simulink model "Analyse_Data_LORD"  (R2019b)
settings: Solver=FixedStepAuto  StartTime=0.0  StopTime=6488  FixedStep=0.01  RelTol=1e-3
settings Model: Creator=ReneB  LastModifiedBy=Rene Budich
settings SFSimCC: CustomCodeUndefinedFunction=UseInterfaceOnly

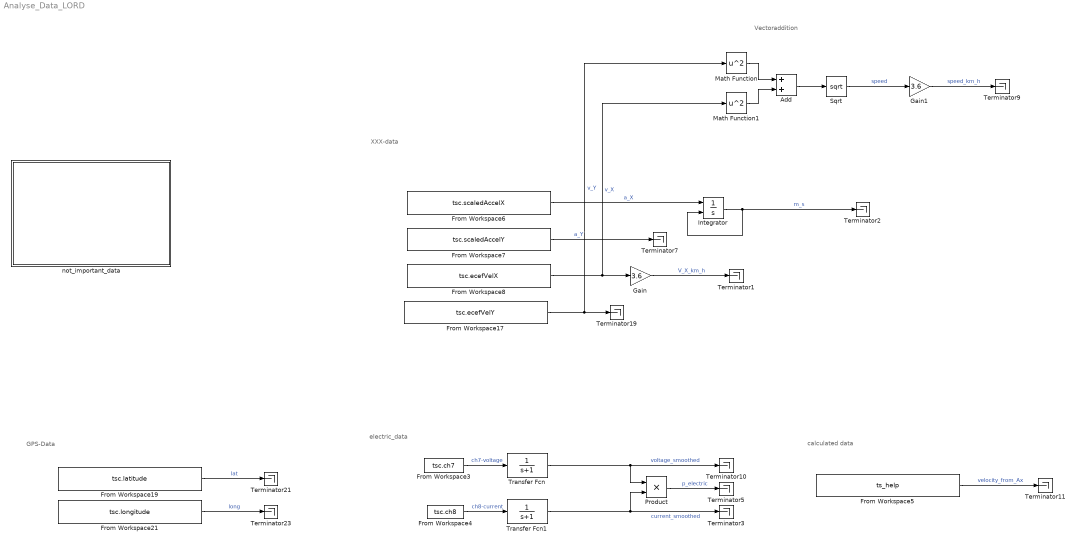
== system Analyse_Data_LORD ==
  note: Vectoraddition
  note: GPS-Data
  note: electric_data
  note: calculated data
  note: XXX-data
  Add : Sum
  From Workspace17 : FromWorkspace  VariableName=tsc.ecefVelY  SampleTime=0
  From Workspace19 : FromWorkspace  VariableName=tsc.latitude  SampleTime=0
  From Workspace21 : FromWorkspace  VariableName=tsc.longitude  SampleTime=0
  From Workspace3 : FromWorkspace  VariableName=tsc.ch7  SampleTime=0
  From Workspace4 : FromWorkspace  VariableName=tsc.ch8  SampleTime=0
  From Workspace5 : FromWorkspace  VariableName=ts_help  SampleTime=0
  From Workspace6 : FromWorkspace  VariableName=tsc.scaledAccelX  SampleTime=0
  From Workspace7 : FromWorkspace  VariableName=tsc.scaledAccelY  SampleTime=0
  From Workspace8 : FromWorkspace  VariableName=tsc.ecefVelX  SampleTime=0
  Gain : Gain  Gain=3.6
  Gain1 : Gain  Gain=3.6
  Integrator : Integrator  InitialConditionSource=external
  Math Function : Math  Operator=square  SignedPower=off  SaturateOnIntegerOverflow=on
  Math Function1 : Math  Operator=square  SignedPower=off  SaturateOnIntegerOverflow=on
  Product : Product
  Sqrt : Sqrt  SaturateOnIntegerOverflow=on
  Terminator{1..3,5,7,9..11,19,21,23} (11 alike) : Terminator
  Transfer Fcn : TransferFcn  Denominator=[1 1]
  Transfer Fcn1 : TransferFcn  Denominator=[1 1]
  not_important_data : Subsystem
  wires:
  From Workspace7/1 -> Terminator7/1  "a_Y"
  From Workspace8/1 -> Math Function1/1, Gain/1  "v_X"
  From Workspace6/1 -> Integrator/1  "a_X"
  From Workspace17/1 -> Math Function/1, Terminator19/1  "v_Y"
  From Workspace19/1 -> Terminator21/1  "lat"
  From Workspace21/1 -> Terminator23/1  "long"
  Gain/1 -> Terminator1/1  "V_X_km_h"
  Integrator/1 -> Integrator/2, Terminator2/1  "m_s"
  From Workspace3/1 -> Transfer Fcn/1  "ch7-voltage"
  From Workspace4/1 -> Transfer Fcn1/1  "ch8-current"
  From Workspace5/1 -> Terminator11/1  "velocity_from_Ax"
  Product/1 -> Terminator5/1  "p_electric"
  Transfer Fcn/1 -> Terminator10/1, Product/1  "voltage_smoothed"
  Transfer Fcn1/1 -> Product/2, Terminator3/1  "current_smoothed"
  Math Function/1 -> Add/1
  Math Function1/1 -> Add/2
  Sqrt/1 -> Gain1/1  "speed"
  Add/1 -> Sqrt/1
  Gain1/1 -> Terminator9/1  "speed_km_h"

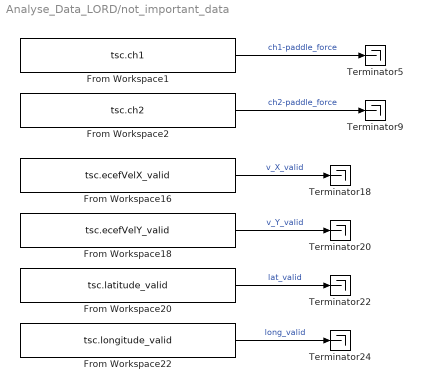
== system Analyse_Data_LORD/not_important_data ==
  From Workspace1 : FromWorkspace  VariableName=tsc.ch1  SampleTime=0
  From Workspace16 : FromWorkspace  VariableName=tsc.ecefVelX_valid  SampleTime=0
  From Workspace18 : FromWorkspace  VariableName=tsc.ecefVelY_valid  SampleTime=0
  From Workspace2 : FromWorkspace  VariableName=tsc.ch2  SampleTime=0
  From Workspace20 : FromWorkspace  VariableName=tsc.latitude_valid  SampleTime=0
  From Workspace22 : FromWorkspace  VariableName=tsc.longitude_valid  SampleTime=0
  Terminator{5,9,18,20,22,24} (6 alike) : Terminator
  wires:
  From Workspace1/1 -> Terminator5/1  "ch1-paddle_force"
  From Workspace18/1 -> Terminator20/1  "v_Y_valid"
  From Workspace2/1 -> Terminator9/1  "ch2-paddle_force"
  From Workspace20/1 -> Terminator22/1  "lat_valid"
  From Workspace16/1 -> Terminator18/1  "v_X_valid"
  From Workspace22/1 -> Terminator24/1  "long_valid"
